simulink model "ModelVerification"  (R2020a)
settings: Solver=VariableStepAuto  StartTime=0.0  StopTime=50  RelTol=1e-3
undefined symbols (not defined in the file): A_ss, B_ss, Bd_ss, c_s, C_ss
libraries: fl_lib x14, nesl_utility x8, simulink x1
settings Model: Creator=juan  LastModifiedBy=juan

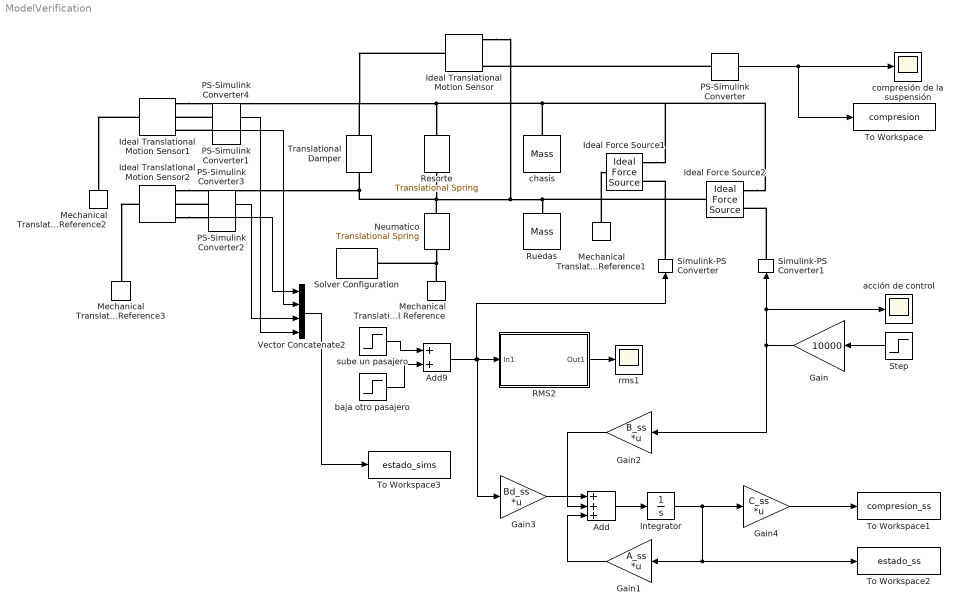
== system ModelVerification ==
  Add : Sum  Inputs=+++
  Add9 : Sum
  Gain : Gain  Gain=10000
  Gain1 : Gain  Gain=A_ss  Multiplication=Matrix(K*u)
  Gain2 : Gain  Gain=B_ss  Multiplication=Matrix(K*u)
  Gain3 : Gain  Gain=Bd_ss  Multiplication=Matrix(K*u)
  Gain4 : Gain  Gain=C_ss  Multiplication=Matrix(K*u)
  Ideal Force Source1 : fl_lib/Mechanical/Mechanical Sources/Ideal Force Source
  Ideal Force Source2 : fl_lib/Mechanical/Mechanical Sources/Ideal Force Source
  Ideal Translational Motion Sensor : fl_lib/Mechanical/Mechanical Sensors/Ideal Translational Motion Sensor  offset=0 m
  Ideal Translational Motion Sensor1 : fl_lib/Mechanical/Mechanical Sensors/Ideal Translational Motion Sensor  offset=0 m
  Ideal Translational Motion Sensor2 : fl_lib/Mechanical/Mechanical Sensors/Ideal Translational Motion Sensor  offset=0 m
  Integrator : Integrator
  Mechanical Translational Reference{,1..3} (4 alike) : fl_lib/Mechanical/Translational Elements/Mechanical Translational Reference
  Neumatico : fl_lib/Mechanical/Translational Elements/Translational Spring  spr_rate=k_t N/m  v_specify=off  v_priority=None  v=0 m/s  v_nominal_specify=off  v_nominal_unit=m/s  v_nominal_value=1  f_specify=off  f_priority=None  f=0 N  f_nominal_specify=off  f_nominal_unit=N  f_nominal_value=1  x_specify=off  x_priority=High  x=0 m  x_nominal_specify=off  x_nominal_unit=m  x_nominal_value=1
  PS-Simulink Converter{,1..4} (5 alike) : nesl_utility/PS-Simulink Converter  PhysicalDomain=network_engine_domain  SubClassName=ps_output  LeftPortType=input  RightPortType=output  PseudoPeriodic=off  Frequencies=[]  Unit=1  AffineConversion=off
  RMS2 : Subsystem
  Resorte : fl_lib/Mechanical/Translational Elements/Translational Spring  spr_rate=k_s N/m  v_specify=off  v_priority=None  v=0 m/s  v_nominal_specify=off  v_nominal_unit=m/s  v_nominal_value=1  f_specify=off  f_priority=None  f=0 N  f_nominal_specify=off  f_nominal_unit=N  f_nominal_value=1  x_specify=off  x_priority=High  x=0 m  x_nominal_specify=off  x_nominal_unit=m  x_nominal_value=1
  Ruedas : fl_lib/Mechanical/Translational Elements/Mass  mass=m_u kg  v_specify=off  v_priority=High  v=0 m/s  v_nominal_specify=off  v_nominal_unit=m/s  v_nominal_value=1  f_specify=off  f_priority=None  f=0 N  f_nominal_specify=off  f_nominal_unit=N  f_nominal_value=1
  Simulink-PS Converter : nesl_utility/Simulink-PS Converter  PhysicalDomain=network_engine_domain  SubClassName=ps_input  LeftPortType=input  RightPortType=output  PseudoPeriodic=off  Frequencies=[]  NoiseDistribution=none  NoiseParameters=[]  Unit=1  AffineConversion=off  FilteringAndDerivatives=provide  SimscapeFilterOrder=1  InputFilterTimeConstant=0.001  UdotUserProvided=0
  Simulink-PS Converter1 : nesl_utility/Simulink-PS Converter  PhysicalDomain=network_engine_domain  SubClassName=ps_input  LeftPortType=input  RightPortType=output  PseudoPeriodic=off  Frequencies=[]  NoiseDistribution=none  NoiseParameters=[]  Unit=1  AffineConversion=off  FilteringAndDerivatives=provide  SimscapeFilterOrder=1  InputFilterTimeConstant=0.001  UdotUserProvided=0
  Solver Configuration : nesl_utility/Solver Configuration  PhysicalDomain=network_engine_domain  SubClassName=solver  LeftPortType=input  RightPortType=generic  Tones=[]  Harmonics=[]  SimulateNoise=off  Profile=off  UseLocalSampling=off  EnableSwitchedLinearOptims=on  FrequencyDomain=off  UseCCode=off  RelTol=0.001  AbsTol=1e-06  MinStep=1e-09  ToWorkspace=off  RevertToSquareIcSolve=off  NumHomotopyIterations=100  PhasorMode=off  PhasorModeNumHarmonics=1  DoDC=off  ResidualTolerance=1e-09  UseLocalSolver=off  LocalSolverChoice=NE_BACKWARD_EULER_ADVANCER  LocalSolverSampleTime=0.001  DoFixedCost=off  MaxNonlinIter=3  MaxModeIter=2  LinearAlgebra=Sparse  EquationFormulation=NE_TIME_EF  DelaysMemoryBudget=1024  AutomaticFiltering=on  FilteringTimeConstant=0.001  PartitionStorageMethod=AS_NEEDED  PartitionMemoryBudget=1024  PartitionMethod=FAST
  Step : Step  SampleTime=0
  To Workspace : ToWorkspace  VariableName=compresion  SaveFormat=Structure With Time  SampleTime=-1
  To Workspace1 : ToWorkspace  VariableName=compresion_ss  SaveFormat=Structure With Time  SampleTime=-1
  To Workspace2 : ToWorkspace  VariableName=estado_ss  SaveFormat=Structure With Time  SampleTime=-1
  To Workspace3 : ToWorkspace  VariableName=estado_sims  SaveFormat=Structure With Time  SampleTime=-1
  Translational Damper : fl_lib/Mechanical/Translational Elements/Translational Damper  D=c_s N/(m/s)  v_specify=off  v_priority=None  v=0 m/s  v_nominal_specify=off  v_nominal_unit=m/s  v_nominal_value=1  f_specify=off  f_priority=None  f=0 N  f_nominal_specify=off  f_nominal_unit=N  f_nominal_value=1
  Vector Concatenate2 : Concatenate  NumInputs=4
  acción de control : Scope
  baja otro pasajero : Step  Time=25  After=-700  SampleTime=0
  chasis : fl_lib/Mechanical/Translational Elements/Mass  mass=m_s kg  v_specify=off  v_priority=High  v=0 m/s  v_nominal_specify=off  v_nominal_unit=m/s  v_nominal_value=1  f_specify=off  f_priority=None  f=0 N  f_nominal_specify=off  f_nominal_unit=N  f_nominal_value=1
  compresión de la suspensión : Scope
  rms1 : Scope
  sube un pasajero : Step  Time=20  After=700  SampleTime=0
  wires:
  PS-Simulink Converter/1 -> To Workspace/1, compresión de la suspensión/1
  baja otro pasajero/1 -> Add9/2
  sube un pasajero/1 -> Add9/1
  RMS2/1(Out1) -> rms1/1
  Step/1 -> Gain/1
  Integrator/1 -> Gain4/1, To Workspace2/1, Gain1/1
  Add/1 -> Integrator/1
  Gain1/1 -> Add/3
  Gain3/1 -> Add/1
  Gain2/1 -> Add/2
  Gain4/1 -> To Workspace1/1
  Gain/1 -> Simulink-PS Converter1/1, acción de control/1, Gain2/1
  Add9/1 -> Simulink-PS Converter/1, Gain3/1, RMS2/1(In1)
  PS-Simulink Converter2/1 -> Vector Concatenate2/1
  PS-Simulink Converter1/1 -> Vector Concatenate2/2
  PS-Simulink Converter3/1 -> Vector Concatenate2/3
  PS-Simulink Converter4/1 -> Vector Concatenate2/4
  Vector Concatenate2/1 -> To Workspace3/1
  connections:
  chasis/LConn1 -- Ideal Force Source1/RConn2 -- Ideal Force Source2/RConn2 -- Resorte/LConn1 -- Translational Damper/LConn1 -- Ideal Translational Motion Sensor/LConn1 -- Ideal Translational Motion Sensor1/RConn1
  Mechanical Translational Reference/LConn1 -- Neumatico/RConn1 -- Solver Configuration/RConn1
  Resorte/RConn1 -- Neumatico/LConn1 -- Ideal Translational Motion Sensor/RConn1 -- Ideal Force Source2/LConn1 -- Ruedas/LConn1 -- Ideal Translational Motion Sensor2/RConn1 -- Translational Damper/RConn1
  PS-Simulink Converter/LConn1 -- Ideal Translational Motion Sensor/RConn3
  Simulink-PS Converter/RConn1 -- Ideal Force Source1/RConn1
  Simulink-PS Converter1/RConn1 -- Ideal Force Source2/RConn1
  Ideal Translational Motion Sensor1/LConn1 -- Mechanical Translational Reference2/LConn1
  Ideal Translational Motion Sensor2/LConn1 -- Mechanical Translational Reference3/LConn1
  PS-Simulink Converter1/LConn1 -- Ideal Translational Motion Sensor1/RConn3
  Ideal Translational Motion Sensor2/RConn3 -- PS-Simulink Converter2/LConn1
  PS-Simulink Converter3/LConn1 -- Ideal Translational Motion Sensor2/RConn2
  PS-Simulink Converter4/LConn1 -- Ideal Translational Motion Sensor1/RConn2
  Mechanical Translational Reference1/LConn1 -- Ideal Force Source1/LConn1

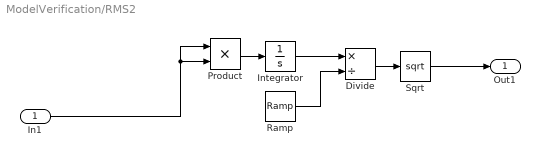
== system ModelVerification/RMS2 ==
  In1 : Inport
  Divide : Product  Inputs=*/
  Integrator : Integrator
  Product : Product
  Ramp : simulink/Sources/Ramp  slope=1  start=0  InitialOutput=0
  Sqrt : Sqrt  SaturateOnIntegerOverflow=on
  Out1 : Outport  VectorParamsAs1DForOutWhenUnconnected=off
  wires:
  Ramp/1 -> Divide/2
  Product/1 -> Integrator/1
  Integrator/1 -> Divide/1
  Sqrt/1 -> Out1/1
  Divide/1 -> Sqrt/1
  In1/1 -> Product/1, Product/2
